simulink model "Fusion_Frame_Model_Architecture"  (R2018a)
settings: Solver=FixedStepAuto  StartTime=0.0  StopTime=SimulationTime  FixedStep=SamplingTime  RelTol=1e-3
undefined symbols (not defined in the file or in its folder): ACTIVATE_CAM, ACTIVATE_RAD, CAM1_detTimeStamp, CAM1_MeasNoise, CAM1_objClassID, CAM1_PX, CAM1_PY, CAM1_VX, CAM1_VY, CAM2_detTimeStamp, CAM2_MeasNoise, CAM2_objClassID, CAM2_PX, CAM2_PY, CAM2_VX, CAM2_VY, CAM3_detTimeStamp, CAM3_MeasNoise, CAM3_objClassID, CAM3_PX, CAM3_PY, CAM3_VX, CAM3_VY, CAM4_detTimeStamp, CAM4_MeasNoise, CAM4_objClassID, CAM4_PX, CAM4_PY, CAM4_VX, CAM4_VY, CAM5_detTimeStamp, CAM5_MeasNoise, CAM5_objClassID, CAM5_PX, CAM5_PY, CAM5_VX, CAM5_VY, CAM6_detTimeStamp, CAM6_MeasNoise, CAM6_objClassID, CAM6_PX, CAM6_PY, CAM6_VX, CAM6_VY, CAM7_detTimeStamp, CAM7_MeasNoise, CAM7_objClassID, CAM7_PX, CAM7_PY, CAM7_VX, CAM7_VY, CAM8_detTimeStamp, CAM8_MeasNoise, CAM8_objClassID, CAM8_PX, CAM8_PY, CAM8_VX, CAM8_VY, CAM_nMeas, CAM_TYPE ... (+181)
libraries: simulink_extras x4
(part 1 of 11)
settings Model: SimulationMode=accelerator  Creator=Udit Bhaskar  LastModifiedBy=Udit Bhaskar
settings OptimizationCC: EfficientMapNaN2IntZero=off
settings HardwareCC: TargetBitPerPointer=64  TargetBitPerSizeT=64  TargetBitPerPtrDiffT=64  TargetLongLongMode=on  TargetIntDivRoundTo=Zero  TargetEndianess=LittleEndian  TargetWordSize=64  TargetHWDeviceType=MATLAB Host  ProdEqTarget=off
settings CodeAppCC: MaxIdLength=128
settings GRTTargetCC: TargetLangStandard=C89/C90 (ANSI)  CombineOutputUpdateFcns=off  GRTInterface=on

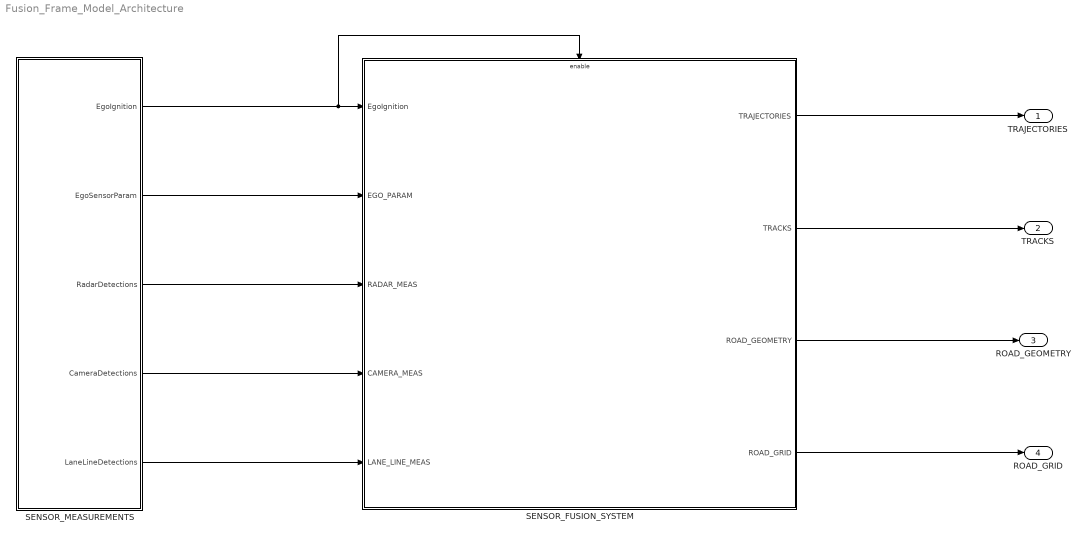
== system Fusion_Frame_Model_Architecture ==
  SENSOR_FUSION_SYSTEM : Subsystem
  SENSOR_MEASUREMENTS : Subsystem
  TRAJECTORIES : Outport
  TRACKS : Outport  Port=2
  ROAD_GEOMETRY : Outport  Port=3
  ROAD_GRID : Outport  Port=4
  wires:
  SENSOR_MEASUREMENTS/2(EgoSensorParam) -> SENSOR_FUSION_SYSTEM/2(EGO_PARAM)
  SENSOR_MEASUREMENTS/3(RadarDetections) -> SENSOR_FUSION_SYSTEM/3(RADAR_MEAS)
  SENSOR_MEASUREMENTS/4(CameraDetections) -> SENSOR_FUSION_SYSTEM/4(CAMERA_MEAS)
  SENSOR_MEASUREMENTS/5(LaneLineDetections) -> SENSOR_FUSION_SYSTEM/5(LANE_LINE_MEAS)
  SENSOR_FUSION_SYSTEM/2(TRACKS) -> TRACKS/1
  SENSOR_FUSION_SYSTEM/4(ROAD_GRID) -> ROAD_GRID/1
  SENSOR_FUSION_SYSTEM/1(TRAJECTORIES) -> TRAJECTORIES/1
  SENSOR_FUSION_SYSTEM/3(ROAD_GEOMETRY) -> ROAD_GEOMETRY/1
  SENSOR_MEASUREMENTS/1(EgoIgnition) -> SENSOR_FUSION_SYSTEM/1(EgoIgnition), SENSOR_FUSION_SYSTEM/Enable

== system Fusion_Frame_Model_Architecture/SENSOR_FUSION_SYSTEM ==
  EgoIgnition : Inport
  EGO_PARAM : Inport  Port=2
  RADAR_MEAS : Inport  Port=3
  CAMERA_MEAS : Inport  Port=4
  LANE_LINE_MEAS : Inport  Port=5
  Enable : EnablePort
  OBJECT_TRACKER_SENSOR_FUSION : Subsystem
  ROAD_GEOMETRY_CAMERA_FUSION : Subsystem
  Terminator : Terminator
  TRAJECTORIES : Outport
  TRACKS : Outport  Port=2
  ROAD_GEOMETRY : Outport  Port=3
  ROAD_GRID : Outport  Port=4
  wires:
  RADAR_MEAS/1 -> OBJECT_TRACKER_SENSOR_FUSION/3(RadCAN)
  LANE_LINE_MEAS/1 -> ROAD_GEOMETRY_CAMERA_FUSION/3(LINE_MEAS)
  OBJECT_TRACKER_SENSOR_FUSION/4(CamParam) -> ROAD_GEOMETRY_CAMERA_FUSION/1(CAM_SNSR_PARAM)
  [ego] -> ROAD_GEOMETRY_CAMERA_FUSION/2(EGO_PARAM)
  EGO_PARAM/1 -> [ego], OBJECT_TRACKER_SENSOR_FUSION/2(EgoData)
  CAMERA_MEAS/1 -> OBJECT_TRACKER_SENSOR_FUSION/4(CamCAN)
  EgoIgnition/1 -> OBJECT_TRACKER_SENSOR_FUSION/1(EgoIgnition)
  OBJECT_TRACKER_SENSOR_FUSION/1("TRAJECTORY_DATA ") -> TRAJECTORIES/1
  OBJECT_TRACKER_SENSOR_FUSION/2(TRACK_DATA) -> TRACKS/1
  ROAD_GEOMETRY_CAMERA_FUSION/1(ROAD_GEOMETRY) -> ROAD_GEOMETRY/1
  ROAD_GEOMETRY_CAMERA_FUSION/2(ROAD_GRID) -> ROAD_GRID/1
  OBJECT_TRACKER_SENSOR_FUSION/3(SENSOR_FOV_GRID) -> Terminator/1

== system Fusion_Frame_Model_Architecture/SENSOR_MEASUREMENTS ==
  RADAR_CAMERA_EGO_SENSOR_INTERFACE : Subsystem
  Subsystem : Subsystem
  Subsystem1 : Subsystem
  EgoIgnition : Outport
  EgoSensorParam : Outport  Port=2
  RadarDetections : Outport  Port=3
  CameraDetections : Outport  Port=4
  LaneLineDetections : Outport  Port=5
  wires:
  RADAR_CAMERA_EGO_SENSOR_INTERFACE/11(C5) -> Subsystem/11(C5)
  RADAR_CAMERA_EGO_SENSOR_INTERFACE/4(R4) -> Subsystem/4(R4)
  RADAR_CAMERA_EGO_SENSOR_INTERFACE/2(R2) -> Subsystem/2(R2)
  RADAR_CAMERA_EGO_SENSOR_INTERFACE/5(R5) -> Subsystem/5(R5)
  RADAR_CAMERA_EGO_SENSOR_INTERFACE/6(R6) -> Subsystem/6(R6)
  RADAR_CAMERA_EGO_SENSOR_INTERFACE/1(R1) -> Subsystem/1(R1)
  Subsystem/1(RadarMeasurementCAN) -> RadarDetections/1
  RADAR_CAMERA_EGO_SENSOR_INTERFACE/9(C3) -> Subsystem/9(C3)
  RADAR_CAMERA_EGO_SENSOR_INTERFACE/8(C2) -> Subsystem/8(C2)
  RADAR_CAMERA_EGO_SENSOR_INTERFACE/3(R3) -> Subsystem/3(R3)
  RADAR_CAMERA_EGO_SENSOR_INTERFACE/13(C7) -> Subsystem/13(C7)
  RADAR_CAMERA_EGO_SENSOR_INTERFACE/7(C1) -> Subsystem/7(C1)
  RADAR_CAMERA_EGO_SENSOR_INTERFACE/10(C4) -> Subsystem/10(C4)
  RADAR_CAMERA_EGO_SENSOR_INTERFACE/12(C6) -> Subsystem/12(C6)
  Subsystem/2(CameraMeasurementCAN) -> CameraDetections/1
  RADAR_CAMERA_EGO_SENSOR_INTERFACE/14(C8) -> Subsystem/14(C8)
  RADAR_CAMERA_EGO_SENSOR_INTERFACE/15(CAM_LINE1) -> Subsystem1/1(CAM_LINE1)
  RADAR_CAMERA_EGO_SENSOR_INTERFACE/16(CAM_LINE2) -> Subsystem1/2(CAM_LINE2)
  RADAR_CAMERA_EGO_SENSOR_INTERFACE/17(CAM_LINE3) -> Subsystem1/3(CAM_LINE3)
  RADAR_CAMERA_EGO_SENSOR_INTERFACE/18(CAM_LINE4) -> Subsystem1/4(CAM_LINE4)
  RADAR_CAMERA_EGO_SENSOR_INTERFACE/19(CAM_LINE5) -> Subsystem1/5(CAM_LINE5)
  RADAR_CAMERA_EGO_SENSOR_INTERFACE/20(CAM_LINE6) -> Subsystem1/6(CAM_LINE6)
  RADAR_CAMERA_EGO_SENSOR_INTERFACE/21(CAM_LINE7) -> Subsystem1/7(CAM_LINE7)
  RADAR_CAMERA_EGO_SENSOR_INTERFACE/22(CAM_LINE8) -> Subsystem1/8(CAM_LINE8)
  Subsystem1/1(LineMeasurementsCAN) -> LaneLineDetections/1
  RADAR_CAMERA_EGO_SENSOR_INTERFACE/23(EGO) -> EgoSensorParam/1
  RADAR_CAMERA_EGO_SENSOR_INTERFACE/24(EgoIgnition) -> EgoIgnition/1

== system Fusion_Frame_Model_Architecture/SENSOR_FUSION_SYSTEM/OBJECT_TRACKER_SENSOR_FUSION ==
  EgoIgnition : Inport
  EgoData : Inport  Port=2
  RadCAN : Inport  Port=3
  CamCAN : Inport  Port=4
  CAMERA_HOMOGENEOUS_FUSION : Subsystem
  RADAR_CAMERA_HETEROGENEOUS_FUSION : Subsystem
  RADAR_HOMOGENEOUS_FUSION : Subsystem
  SENSOR_LAYOUT_AND_CHRACTERIZATION : Subsystem
  SPATIAL_ALLIGNMENT1 : Subsystem
  TRACKS_TRAJECTORY_COMPUTATION : Subsystem
  Unit Delay : UnitDelay  InitialCondition=false  SampleTime=-1
  "TRAJECTORY_DATA " : Outport
  TRACK_DATA : Outport  Port=2
  SENSOR_FOV_GRID : Outport  Port=3
  CamParam : Outport  Port=4
  wires:
  EgoData/1 -> TRACKS_TRAJECTORY_COMPUTATION/2(EGO_DATA)
  SPATIAL_ALLIGNMENT1/1(RadarMeasTransformed) -> RADAR_HOMOGENEOUS_FUSION/3(RADAR_MEAS)
  RadCAN/1 -> SPATIAL_ALLIGNMENT1/3(RadarCAN)
  SPATIAL_ALLIGNMENT1/2(CameraMeasTransformed) -> CAMERA_HOMOGENEOUS_FUSION/2(CAMERA_MEAS)
  CamCAN/1 -> SPATIAL_ALLIGNMENT1/4(CameraCAN)
  SENSOR_LAYOUT_AND_CHRACTERIZATION/1(RAD_SNSR_PARAM) -> SPATIAL_ALLIGNMENT1/1(RadarCallibrationParam), [RAD_PARAM]
  SENSOR_LAYOUT_AND_CHRACTERIZATION/2(CAM_SNSR_PARAM) -> SPATIAL_ALLIGNMENT1/2(CameraCallibrationParam), [CAM_PARAM]
  SENSOR_LAYOUT_AND_CHRACTERIZATION/3(GRID_CHARACTERIZATION) -> [GRID]
  EgoIgnition/1 -> Unit Delay/1
  Unit Delay/1 -> SENSOR_LAYOUT_AND_CHRACTERIZATION/Trigger
  [GRID] -> CAMERA_HOMOGENEOUS_FUSION/1(GRID), RADAR_HOMOGENEOUS_FUSION/4(GRID)
  RADAR_HOMOGENEOUS_FUSION/1(RADAR_TRACKS_FUS) -> RADAR_CAMERA_HETEROGENEOUS_FUSION/1(RADAR_TRACKS_FUS), RADAR_HOMOGENEOUS_FUSION/1(RADAR_TRACKS_PREV)
  CAMERA_HOMOGENEOUS_FUSION/1(CAMERA_TRACKS_FUS) -> RADAR_CAMERA_HETEROGENEOUS_FUSION/2(CAMERA_TRACKS_FUS), CAMERA_HOMOGENEOUS_FUSION/4(CAMERA_TRACKS_PREV)
  TRACKS_TRAJECTORY_COMPUTATION/1(TRAJECTORY) -> "TRAJECTORY_DATA "/1, TRACKS_TRAJECTORY_COMPUTATION/1(TRAJECTORIES_PREV)
  [RAD_PARAM] -> RADAR_HOMOGENEOUS_FUSION/2(RAD_PARAM)
  [CAM_PARAM] -> CAMERA_HOMOGENEOUS_FUSION/3(CAM_PARAM)
  RADAR_CAMERA_HETEROGENEOUS_FUSION/1(FUS_TRACKS) -> TRACKS_TRAJECTORY_COMPUTATION/3(RAD_CAM_TRACKS_FUS), TRACK_DATA/1, RADAR_CAMERA_HETEROGENEOUS_FUSION/3(RAD_CAM_TRACKS_PREV)
  [GRID] -> SENSOR_FOV_GRID/1
  [CAM_PARAM] -> CamParam/1

== system Fusion_Frame_Model_Architecture/SENSOR_FUSION_SYSTEM/ROAD_GEOMETRY_CAMERA_FUSION ==
  CAM_SNSR_PARAM : Inport
  EGO_PARAM : Inport  Port=2
  LINE_MEAS : Inport  Port=3
  EGO_LANE_CENTER_LINE_ESTIMATION_FROM_LEFT_BOUNDARY : Subsystem
  EGO_LANE_CENTER_LINE_ESTIMATION_FROM_RIGHT_BOUNDARY : Subsystem
  EGO_LANE_CENTER_LINE_HYPOTHESIS_FUSION : Subsystem
  EGO_LANE_LEFT_BOUNDARY_LINE_FUSION : Subsystem
  EGO_LANE_RIGHT_BOUNDARY_LINE_FUSION : Subsystem
  EGO_LANE_WIDTH_ESTIMATION : Subsystem
  ROAD_GEOMERY_AND_GRID_COMPUTATION : Subsystem
  SPATIAL_ALLIGNMENT_CLOTHOID_COEFFICIENTS : Subsystem
  ROAD_GEOMETRY : Outport
  ROAD_GRID : Outport  Port=2
  wires:
  LINE_MEAS/1 -> SPATIAL_ALLIGNMENT_CLOTHOID_COEFFICIENTS/2(LINE_CLOTHOID_MEASUREMENTS)
  EGO_LANE_LEFT_BOUNDARY_LINE_FUSION/1(EGO_LANE_LEFT_LINE_TRACK) -> EGO_LANE_WIDTH_ESTIMATION/2(EGO_LANE_RIGHT_LINE_TRACK), EGO_LANE_LEFT_BOUNDARY_LINE_FUSION/1(EGO_LANE_LEFT_LINE_TRACK_prev), EGO_LANE_CENTER_LINE_ESTIMATION_FROM_LEFT_BOUNDARY/2(EGO_LANE_LEFT_LINE_TRACK)
  EGO_LANE_CENTER_LINE_HYPOTHESIS_FUSION/1(EGO_LANE_CENTER_LINE_CURR) -> ROAD_GEOMERY_AND_GRID_COMPUTATION/2(EGO_LANE_CENTER_LINE_TRACK)
  CAM_SNSR_PARAM/1 -> SPATIAL_ALLIGNMENT_CLOTHOID_COEFFICIENTS/1(CAM_SENSOR_PARAM)
  SPATIAL_ALLIGNMENT_CLOTHOID_COEFFICIENTS/1(LEFT_LINE_MEAS) -> EGO_LANE_LEFT_BOUNDARY_LINE_FUSION/2(EGO_LANE_LEFT_LINE_MEAS)
  EGO_LANE_RIGHT_BOUNDARY_LINE_FUSION/1(EGO_LANE_RIGHT_LINE_TRACK) -> EGO_LANE_WIDTH_ESTIMATION/3(EGO_LANE_LEFT_LINE_TRACK), EGO_LANE_CENTER_LINE_ESTIMATION_FROM_RIGHT_BOUNDARY/2(EGO_LANE_RIGHT_LINE_TRACK), EGO_LANE_RIGHT_BOUNDARY_LINE_FUSION/2(EGO_LANE_RIGHT_LINE_TRACK_prev)
  EGO_LANE_WIDTH_ESTIMATION/1(EGO_LANE_WIDTH) -> EGO_LANE_WIDTH_ESTIMATION/1(EGO_LANE_WIDTH_prev), EGO_LANE_CENTER_LINE_ESTIMATION_FROM_LEFT_BOUNDARY/3(EGO_LANE_WIDTH), EGO_LANE_CENTER_LINE_ESTIMATION_FROM_RIGHT_BOUNDARY/1(EGO_LANE_WIDTH), [WIDTH]
  EGO_LANE_CENTER_LINE_ESTIMATION_FROM_LEFT_BOUNDARY/1(EGO_LANE_CENTER_LINE_TRACK_HYP1) -> EGO_LANE_CENTER_LINE_HYPOTHESIS_FUSION/1(EGO_LANE_CENTER_LINE_HYP1)
  ROAD_GEOMERY_AND_GRID_COMPUTATION/2(ROAD_GRID) -> ROAD_GRID/1, ROAD_GEOMERY_AND_GRID_COMPUTATION/4(ROAD_GRID_prev)
  EGO_PARAM/1 -> [EGO_PARAM]
  [WIDTH] -> ROAD_GEOMERY_AND_GRID_COMPUTATION/1(EGO_LANE_WIDTH)
  [EGO_PARAM] -> ROAD_GEOMERY_AND_GRID_COMPUTATION/3(EGO_PARAM)
  ROAD_GEOMERY_AND_GRID_COMPUTATION/1(ROAD_GEOMETRY) -> ROAD_GEOMETRY/1
  SPATIAL_ALLIGNMENT_CLOTHOID_COEFFICIENTS/2("RIGHT_LINE_MEAS ") -> EGO_LANE_RIGHT_BOUNDARY_LINE_FUSION/1(EGO_LANE_RIGHT_LINE_MEAS)
  EGO_LANE_CENTER_LINE_ESTIMATION_FROM_RIGHT_BOUNDARY/1(EGO_LANE_CENTER_LINE_TRACK_HYP2) -> EGO_LANE_CENTER_LINE_HYPOTHESIS_FUSION/2(EGO_LANE_CENTER_LINE_HYP2)
  EGO_LANE_CENTER_LINE_HYPOTHESIS_FUSION/2(EGO_LANE_CENTER_LINE_PRED) -> EGO_LANE_CENTER_LINE_ESTIMATION_FROM_RIGHT_BOUNDARY/3(EGO_LANE_CENTER_LINE_TRACK_pred), EGO_LANE_CENTER_LINE_ESTIMATION_FROM_LEFT_BOUNDARY/1(EGO_LANE_CENTER_LINE_TRACK_pred)

== system Fusion_Frame_Model_Architecture/SENSOR_MEASUREMENTS/RADAR_CAMERA_EGO_SENSOR_INTERFACE ==
  CameraSensors : Subsystem
  Clock : Subsystem
  EgoSensors : Subsystem
  Ground{,1..3} (4 alike) : Ground
  RadarSensors : Subsystem
  RoadSensors : Subsystem
  R1 : Outport
  R2 : Outport  Port=2
  R3 : Outport  Port=3
  R4 : Outport  Port=4
  R5 : Outport  Port=5
  R6 : Outport  Port=6
  C1 : Outport  Port=7
  C2 : Outport  Port=8
  C3 : Outport  Port=9
  C4 : Outport  Port=10
  C5 : Outport  Port=11
  C6 : Outport  Port=12
  C7 : Outport  Port=13
  C8 : Outport  Port=14
  CAM_LINE1 : Outport  Port=15
  CAM_LINE2 : Outport  Port=16
  CAM_LINE3 : Outport  Port=17
  CAM_LINE4 : Outport  Port=18
  CAM_LINE5 : Outport  Port=19
  CAM_LINE6 : Outport  Port=20
  CAM_LINE7 : Outport  Port=21
  CAM_LINE8 : Outport  Port=22
  EGO : Outport  Port=23
  EgoIgnition : Outport  Port=24
  wires:
  RadarSensors/6(R6) -> R6/1
  RadarSensors/4(R4) -> R4/1
  Clock/2(nObjRadar) -> RadarSensors/2(nObjRadar)
  Clock/3(nObjCamera) -> CameraSensors/2(nObjCamera)
  CameraSensors/3(C3) -> C3/1
  RadarSensors/5(R5) -> R5/1
  CameraSensors/5(C5) -> C5/1
  CameraSensors/4(C4) -> C4/1
  CameraSensors/8(C8) -> C8/1
  CameraSensors/7(C7) -> C7/1
  CameraSensors/6(C6) -> C6/1
  CameraSensors/2(C2) -> C2/1
  RadarSensors/2(R2) -> R2/1
  RadarSensors/3(R3) -> R3/1
  CameraSensors/1(C1) -> C1/1
  RadarSensors/1(R1) -> R1/1
  Clock/1(time) -> CameraSensors/1(time), RoadSensors/1(time), EgoSensors/1(timeIdx), RadarSensors/1(time)
  Clock/4(nLinesCamera) -> RoadSensors/2(nLinesCamera)
  RoadSensors/1(C1) -> CAM_LINE1/1
  RoadSensors/2(C2) -> CAM_LINE2/1
  RoadSensors/3(C3) -> CAM_LINE3/1
  RoadSensors/4(C4) -> CAM_LINE4/1
  RoadSensors/5(C5) -> CAM_LINE5/1
  RoadSensors/6(C6) -> CAM_LINE6/1
  RoadSensors/7(C7) -> CAM_LINE7/1
  RoadSensors/8(C8) -> CAM_LINE8/1
  EgoSensors/1(EgoSensorData) -> EGO/1
  Ground1/1 -> RadarSensors/3(RADSensorBUS)
  Ground2/1 -> CameraSensors/3(CAMSensorBUS)
  Ground/1 -> EgoSensors/2(In1)
  Ground3/1 -> RoadSensors/3(CameraLineCoeff1)
  EgoSensors/2(EgoIgnitionStatus) -> EgoIgnition/1

== system Fusion_Frame_Model_Architecture/SENSOR_MEASUREMENTS/Subsystem ==
  R1 : Inport
  R2 : Inport  Port=2
  R3 : Inport  Port=3
  R4 : Inport  Port=4
  R5 : Inport  Port=5
  R6 : Inport  Port=6
  C1 : Inport  Port=7
  C2 : Inport  Port=8
  C3 : Inport  Port=9
  C4 : Inport  Port=10
  C5 : Inport  Port=11
  C6 : Inport  Port=12
  C7 : Inport  Port=13
  C8 : Inport  Port=14
  Bus Creator : BusCreator  Inputs=6  OutDataTypeStr=Bus: RAD_MEAS_INTERFACE  NonVirtualBus=on
      settings: InheritFromInputs=off
  Bus Creator1 : BusCreator  Inputs=8  OutDataTypeStr=Bus: CAM_MEAS_INTERFACE  NonVirtualBus=on
      settings: InheritFromInputs=off
  RadarMeasurementCAN : Outport
  CameraMeasurementCAN : Outport  Port=2
  wires:
  R1/1 -> Bus Creator/1  "R1"
  R6/1 -> Bus Creator/6  "R6"
  R5/1 -> Bus Creator/5  "R5"
  R4/1 -> Bus Creator/4  "R4"
  R3/1 -> Bus Creator/3  "R3"
  R2/1 -> Bus Creator/2  "R2"
  Bus Creator/1 -> RadarMeasurementCAN/1
  C1/1 -> Bus Creator1/1  "C1"
  C2/1 -> Bus Creator1/2  "C2"
  C3/1 -> Bus Creator1/3  "C3"
  C4/1 -> Bus Creator1/4  "C4"
  C5/1 -> Bus Creator1/5  "C5"
  C6/1 -> Bus Creator1/6  "C6"
  C7/1 -> Bus Creator1/7  "C7"
  C8/1 -> Bus Creator1/8  "C8"
  Bus Creator1/1 -> CameraMeasurementCAN/1

== system Fusion_Frame_Model_Architecture/SENSOR_MEASUREMENTS/Subsystem1 ==
  CAM_LINE1 : Inport
  CAM_LINE2 : Inport  Port=2
  CAM_LINE3 : Inport  Port=3
  CAM_LINE4 : Inport  Port=4
  CAM_LINE5 : Inport  Port=5
  CAM_LINE6 : Inport  Port=6
  CAM_LINE7 : Inport  Port=7
  CAM_LINE8 : Inport  Port=8
  Bus Creator : BusCreator  Inputs=8  OutDataTypeStr=Bus: LINE_MEAS_INTERFACE  NonVirtualBus=on
      settings: InheritFromInputs=off
  LineMeasurementsCAN : Outport
  wires:
  CAM_LINE1/1 -> Bus Creator/1  "C1_LINE"
  CAM_LINE2/1 -> Bus Creator/2  "C2_LINE"
  CAM_LINE3/1 -> Bus Creator/3  "C3_LINE"
  CAM_LINE4/1 -> Bus Creator/4  "C4_LINE"
  CAM_LINE5/1 -> Bus Creator/5  "C5_LINE"
  CAM_LINE6/1 -> Bus Creator/6  "C6_LINE"
  CAM_LINE7/1 -> Bus Creator/7  "C7_LINE"
  CAM_LINE8/1 -> Bus Creator/8  "C8_LINE"
  Bus Creator/1 -> LineMeasurementsCAN/1

== system Fusion_Frame_Model_Architecture/SENSOR_FUSION_SYSTEM/OBJECT_TRACKER_SENSOR_FUSION/CAMERA_HOMOGENEOUS_FUSION ==
  GRID : Inport
  CAMERA_MEAS : Inport  Port=2
  CAM_PARAM : Inport  Port=3
  CAMERA_TRACKS_PREV : Inport  Port=4
  DATA_ASSOCIATION_AND_ESTIMATION : Subsystem
  GATING : Subsystem
  NEAREST_NEIGHBOUR_CLUSTERING_FOR_CAMERA_MEASUREMENT : Subsystem
  STATE_PREDICTION : Subsystem
  TRACK_MANAGER : Subsystem
  CAMERA_TRACKS_FUS : Outport
  wires:
  CAMERA_MEAS/1 -> GATING/1(MEAS), [CAM_MEAS], NEAREST_NEIGHBOUR_CLUSTERING_FOR_CAMERA_MEASUREMENT/1(CAMERA_MEAS)
  NEAREST_NEIGHBOUR_CLUSTERING_FOR_CAMERA_MEASUREMENT/1(CAMERA_CLUSTERS) -> GATING/2(CAMERA_CLUSTERS)
  DATA_ASSOCIATION_AND_ESTIMATION/1(TrackParamUpd) -> TRACK_MANAGER/1(TrackParamIn)
  STATE_PREDICTION/1(TrackParamPred) -> GATING/4(TrackParamPred), DATA_ASSOCIATION_AND_ESTIMATION/5(TrackParamPred)
  [unGatedClstr] -> TRACK_MANAGER/2(UnGatedClusters)
  GATING/1(GatedMeasFlag) -> DATA_ASSOCIATION_AND_ESTIMATION/1(GatedMeasFlag)
  GRID/1 -> TRACK_MANAGER/3(Grid)
  GATING/2(GatedMeasLogLikelihood) -> DATA_ASSOCIATION_AND_ESTIMATION/2(MeasLogLikelihood)
  [CAM_MEAS] -> DATA_ASSOCIATION_AND_ESTIMATION/3(Meas)
  GATING/3(UnGatedMeasCluster) -> [unGatedClstr]
  CAMERA_TRACKS_PREV/1 -> STATE_PREDICTION/1(TrackParamPrev)
  TRACK_MANAGER/1(TrackParamUpd) -> CAMERA_TRACKS_FUS/1
  CAM_PARAM/1 -> [CAM_PARAM]
  [CAM_PARAM] -> GATING/3(CAM_PARAM)
  [CAM_PARAM] -> DATA_ASSOCIATION_AND_ESTIMATION/4(CAM_PARAM)

== system Fusion_Frame_Model_Architecture/SENSOR_FUSION_SYSTEM/OBJECT_TRACKER_SENSOR_FUSION/RADAR_CAMERA_HETEROGENEOUS_FUSION ==
  RADAR_TRACKS_FUS : Inport
  CAMERA_TRACKS_FUS : Inport  Port=2
  RAD_CAM_TRACKS_PREV : Inport  Port=3
  FORM_TRACK_GROUPS : Subsystem
  STATE_PREDICTION : Subsystem
  TRACK_MANAGER : Subsystem
  TRACK_TO_TRACK_FUSION : Subsystem
  FUS_TRACKS : Outport
  wires:
  RAD_CAM_TRACKS_PREV/1 -> [RAD_TRACKS], STATE_PREDICTION/1(RAD_CAM_TRACKS_PREV)
  STATE_PREDICTION/1(RAD_CAM_TRACKS_PRED) -> FORM_TRACK_GROUPS/2(RAD_CAM_FUSED_TRACKS), [FUSED_TRACKS]
  CAMERA_TRACKS_FUS/1 -> [CAM_TRACKS], FORM_TRACK_GROUPS/3(CAM_TRACKS)
  RADAR_TRACKS_FUS/1 -> FORM_TRACK_GROUPS/1(RAD_TRACKS)
  FORM_TRACK_GROUPS/1(GROUPED_TRACKS_IDs) -> TRACK_TO_TRACK_FUSION/1(GROUPED_TRACKS_IDs)
  TRACK_TO_TRACK_FUSION/1(RAD_CAM_FUSED_TRACKS_UPD) -> TRACK_MANAGER/1(RAD_CAM_FUSED_TRACKS)
  [CAM_TRACKS] -> TRACK_TO_TRACK_FUSION/3(CAM_TRACKS)
  [RAD_TRACKS] -> TRACK_TO_TRACK_FUSION/2(RAD_TRACKS)
  [FUSED_TRACKS] -> TRACK_TO_TRACK_FUSION/4(RAD_CAM_FUSED_TRACKS_PRED)
  [RAD_TRACKS] -> TRACK_MANAGER/2(RAD_TRACKS)
  [CAM_TRACKS] -> TRACK_MANAGER/3(CAM_TRACKS)
  TRACK_MANAGER/1(RAD_CAM_TRACKS_FUS) -> FUS_TRACKS/1

== system Fusion_Frame_Model_Architecture/SENSOR_FUSION_SYSTEM/OBJECT_TRACKER_SENSOR_FUSION/RADAR_HOMOGENEOUS_FUSION ==
  RADAR_TRACKS_PREV : Inport
  RAD_PARAM : Inport  Port=2
  RADAR_MEAS : Inport  Port=3
  GRID : Inport  Port=4
  DATA_ASSOCIATION_AND_ESTIMATION : Subsystem
  GATING : Subsystem
  SEGREGATE_CLUSTER : Subsystem
  SIMPLYFIED_DBSCAN_FOR_RADAR_MEASUREMENT_GROUPING : Subsystem
  STATE_PREDICTION : Subsystem
  TRACK_MANAGER : Subsystem
  RADAR_TRACKS_FUS : Outport
  wires:
  GRID/1 -> TRACK_MANAGER/3(Grid)
  RADAR_MEAS/1 -> SEGREGATE_CLUSTER/1(RADAR_MEAS), SIMPLYFIED_DBSCAN_FOR_RADAR_MEASUREMENT_GROUPING/1(RADAR_MEAS)
  SIMPLYFIED_DBSCAN_FOR_RADAR_MEASUREMENT_GROUPING/1(RADAR_CLUSTERS) -> SEGREGATE_CLUSTER/2(RADAR_CLUSTERS), GATING/3(RADAR_CLUSTERS)
  SEGREGATE_CLUSTER/1(RADAR_CLSTR_MEAS) -> GATING/1(MEAS), [RAD_MEAS]
  GATING/1(GatedMeasFlag) -> DATA_ASSOCIATION_AND_ESTIMATION/1(GatedMeasFlag)
  STATE_PREDICTION/1(TrackParamPred) -> GATING/4(TrackParamPred), DATA_ASSOCIATION_AND_ESTIMATION/5(TrackParamPred)
  GATING/2(GatedMeasLogLikelihood) -> DATA_ASSOCIATION_AND_ESTIMATION/2(MeasLogLikelihood)
  [RAD_MEAS] -> DATA_ASSOCIATION_AND_ESTIMATION/3(Meas)
  GATING/3(UnGatedMeasCluster) -> [unGatedClstr]
  DATA_ASSOCIATION_AND_ESTIMATION/1(TrackParamUpd) -> TRACK_MANAGER/1(TrackParamIn)
  [unGatedClstr] -> TRACK_MANAGER/2(UnGatedClusters)
  TRACK_MANAGER/1(TrackParamUpd) -> RADAR_TRACKS_FUS/1
  RAD_PARAM/1 -> [RAD_PARAM]
  [RAD_PARAM] -> GATING/2(RAD_PARAM)
  [RAD_PARAM] -> DATA_ASSOCIATION_AND_ESTIMATION/4(RAD_PARAM)
  RADAR_TRACKS_PREV/1 -> STATE_PREDICTION/1(TrackParamPrev)

== system Fusion_Frame_Model_Architecture/SENSOR_FUSION_SYSTEM/OBJECT_TRACKER_SENSOR_FUSION/SENSOR_LAYOUT_AND_CHRACTERIZATION ==
  Trigger : TriggerPort  VariantControl=Variant  PortDimensions=1
  Ground1 : Ground
  Ground2 : Ground
  PRE_COMPUTE_SENSOR_FOV_GRID : Subsystem
  SET_SENSOR_CALLIBRATION_PARAMETER : Subsystem
  RAD_SNSR_PARAM : Outport
  CAM_SNSR_PARAM : Outport  Port=2
  GRID_CHARACTERIZATION : Outport  Port=3
  wires:
  SET_SENSOR_CALLIBRATION_PARAMETER/2(CameraCalibParamUpd) -> CAM_SNSR_PARAM/1, PRE_COMPUTE_SENSOR_FOV_GRID/2(CAMSnsrParam)
  Ground2/1 -> SET_SENSOR_CALLIBRATION_PARAMETER/2(RADSnsrParam)
  Ground1/1 -> SET_SENSOR_CALLIBRATION_PARAMETER/1(CamCalibParam)
  SET_SENSOR_CALLIBRATION_PARAMETER/1(RadarCalibParamUpd) -> RAD_SNSR_PARAM/1, PRE_COMPUTE_SENSOR_FOV_GRID/1(RADSnsrParam)
  PRE_COMPUTE_SENSOR_FOV_GRID/1(GRID_CHARACTERIZATION) -> GRID_CHARACTERIZATION/1

== system Fusion_Frame_Model_Architecture/SENSOR_FUSION_SYSTEM/OBJECT_TRACKER_SENSOR_FUSION/SPATIAL_ALLIGNMENT1 ==
  RadarCallibrationParam : Inport
  CameraCallibrationParam : Inport  Port=2
  RadarCAN : Inport  Port=3
  CameraCAN : Inport  Port=4
  CAMERA_MEASUREMENTS_SPATIAL_ALLIGNMENT : Subsystem
  GET_CAM_MEAS : Subsystem
  GET_RAD_MEAS : Subsystem
  RADAR_MEASUREMENTS_SPATIAL_ALLIGNMENT : Subsystem
  RadarMeasTransformed : Outport
  CameraMeasTransformed : Outport  Port=2
  wires:
  RadarCAN/1 -> GET_RAD_MEAS/2(RadarMeas)
  CameraCAN/1 -> GET_CAM_MEAS/2(CameraMeas)
  GET_CAM_MEAS/2(<C1>) -> CAMERA_MEASUREMENTS_SPATIAL_ALLIGNMENT/2(C1)
  GET_CAM_MEAS/3(<C2>) -> CAMERA_MEASUREMENTS_SPATIAL_ALLIGNMENT/3(C2)
  GET_CAM_MEAS/4(<C3>) -> CAMERA_MEASUREMENTS_SPATIAL_ALLIGNMENT/4(C3)
  GET_CAM_MEAS/5(<C4>) -> CAMERA_MEASUREMENTS_SPATIAL_ALLIGNMENT/5(C4)
  GET_CAM_MEAS/6(<C5>) -> CAMERA_MEASUREMENTS_SPATIAL_ALLIGNMENT/6(C5)
  GET_CAM_MEAS/7(<C6>) -> CAMERA_MEASUREMENTS_SPATIAL_ALLIGNMENT/7(C6)
  GET_CAM_MEAS/8(<C7>) -> CAMERA_MEASUREMENTS_SPATIAL_ALLIGNMENT/8(C7)
  GET_CAM_MEAS/9(<C8>) -> CAMERA_MEASUREMENTS_SPATIAL_ALLIGNMENT/9(C8)
  GET_RAD_MEAS/2(<R1>) -> RADAR_MEASUREMENTS_SPATIAL_ALLIGNMENT/2(R1)
  GET_RAD_MEAS/3(<R2>) -> RADAR_MEASUREMENTS_SPATIAL_ALLIGNMENT/3(R2)
  GET_RAD_MEAS/4(<R3>) -> RADAR_MEASUREMENTS_SPATIAL_ALLIGNMENT/4(R3)
  GET_RAD_MEAS/5(<R4>) -> RADAR_MEASUREMENTS_SPATIAL_ALLIGNMENT/5(R4)
  GET_RAD_MEAS/6(<R5>) -> RADAR_MEASUREMENTS_SPATIAL_ALLIGNMENT/6(R5)
  GET_RAD_MEAS/7(<R6>) -> RADAR_MEASUREMENTS_SPATIAL_ALLIGNMENT/7(R6)
  GET_RAD_MEAS/1(SnsrParam) -> RADAR_MEASUREMENTS_SPATIAL_ALLIGNMENT/1(RadarCalibParam)
  RadarCallibrationParam/1 -> GET_RAD_MEAS/1(RadarParam)
  GET_CAM_MEAS/1(SnsrParam) -> CAMERA_MEASUREMENTS_SPATIAL_ALLIGNMENT/1(CameraCalibParam)
  CameraCallibrationParam/1 -> GET_CAM_MEAS/1(CameraParam)
  CAMERA_MEASUREMENTS_SPATIAL_ALLIGNMENT/1(CameraMeasTransformed) -> CameraMeasTransformed/1
  RADAR_MEASUREMENTS_SPATIAL_ALLIGNMENT/1(RadarMeasTransformed) -> RadarMeasTransformed/1

== system Fusion_Frame_Model_Architecture/SENSOR_FUSION_SYSTEM/OBJECT_TRACKER_SENSOR_FUSION/TRACKS_TRAJECTORY_COMPUTATION ==
  TRAJECTORIES_PREV : Inport
  EGO_DATA : Inport  Port=2
  RAD_CAM_TRACKS_FUS : Inport  Port=3
  EGO_COMPENSATE_TRAJECTORY_HISTORY_BUFFER : Subsystem
  UPDATE_TRAJECTORY_BUFFER_WITH_CURRENT_TRACK_DATA : Subsystem
  TRAJECTORY : Outport
  wires:
  EGO_DATA/1 -> EGO_COMPENSATE_TRAJECTORY_HISTORY_BUFFER/1(RAD_CAM_TRACKS_FUS)
  RAD_CAM_TRACKS_FUS/1 -> UPDATE_TRAJECTORY_BUFFER_WITH_CURRENT_TRACK_DATA/1(RAD_CAM_TRACKS_FUS)
  TRAJECTORIES_PREV/1 -> UPDATE_TRAJECTORY_BUFFER_WITH_CURRENT_TRACK_DATA/2(TRAJECTORIES)
  UPDATE_TRAJECTORY_BUFFER_WITH_CURRENT_TRACK_DATA/1(TRAJECTORIES_UPD) -> EGO_COMPENSATE_TRAJECTORY_HISTORY_BUFFER/2(TRAJECTORIES)
  EGO_COMPENSATE_TRAJECTORY_HISTORY_BUFFER/1(TRAJECTORIES_UPD) -> TRAJECTORY/1

== system Fusion_Frame_Model_Architecture/SENSOR_FUSION_SYSTEM/ROAD_GEOMETRY_CAMERA_FUSION/EGO_LANE_CENTER_LINE_ESTIMATION_FROM_LEFT_BOUNDARY ==
  EGO_LANE_CENTER_LINE_TRACK_pred : Inport
  EGO_LANE_LEFT_LINE_TRACK : Inport  Port=2
  EGO_LANE_WIDTH : Inport  Port=3
  CURVE_FITTING_BY_LEAST_SQUARES : Subsystem
  GENERATE_POINTS_AT_EGO_LANE_CENTER : Subsystem
  INTERPOLATE_POINTS_ALONG_THE_LINE : Subsystem
  KALMAN_FILTER_STATE_UPDATE : Subsystem
  POLYNOMIAL_TO_CLOTHOID_CONVERSION : Subsystem
  EGO_LANE_CENTER_LINE_TRACK_HYP1 : Outport
  wires:
  EGO_LANE_LEFT_LINE_TRACK/1 -> INTERPOLATE_POINTS_ALONG_THE_LINE/1(LEFT_LINE_TRACK)
  EGO_LANE_WIDTH/1 -> GENERATE_POINTS_AT_EGO_LANE_CENTER/2(EgoLaneWidth)
  EGO_LANE_CENTER_LINE_TRACK_pred/1 -> KALMAN_FILTER_STATE_UPDATE/2(CenterLinePred)
  INTERPOLATE_POINTS_ALONG_THE_LINE/1(PointsAlongTheLine) -> GENERATE_POINTS_AT_EGO_LANE_CENTER/1(PointsAlongTheLine)
  GENERATE_POINTS_AT_EGO_LANE_CENTER/1(PointsAlongEgoLaneCenter) -> CURVE_FITTING_BY_LEAST_SQUARES/1(Points)
  CURVE_FITTING_BY_LEAST_SQUARES/1(PolynomialCoefficients) -> POLYNOMIAL_TO_CLOTHOID_CONVERSION/1(PolynomialCoefficients)
  POLYNOMIAL_TO_CLOTHOID_CONVERSION/1(ClothoidCoefficients) -> KALMAN_FILTER_STATE_UPDATE/1(CenterLineHypothesis)
  KALMAN_FILTER_STATE_UPDATE/1(CenterLineHypUpd) -> EGO_LANE_CENTER_LINE_TRACK_HYP1/1

== system Fusion_Frame_Model_Architecture/SENSOR_FUSION_SYSTEM/ROAD_GEOMETRY_CAMERA_FUSION/EGO_LANE_CENTER_LINE_ESTIMATION_FROM_RIGHT_BOUNDARY ==
  EGO_LANE_WIDTH : Inport
  EGO_LANE_RIGHT_LINE_TRACK : Inport  Port=2
  EGO_LANE_CENTER_LINE_TRACK_pred : Inport  Port=3
  CURVE_FITTING_BY_LEAST_SQUARES : Subsystem
  GENERATE_POINTS_AT_EGO_LANE_CENTER : Subsystem
  INTERPOLATE_POINTS_ALONG_THE_LINE : Subsystem
  KALMAN_FILTER_STATE_UPDATE : Subsystem
  POLYNOMIAL_TO_CLOTHOID_CONVERSION : Subsystem
  EGO_LANE_CENTER_LINE_TRACK_HYP2 : Outport
  wires:
  INTERPOLATE_POINTS_ALONG_THE_LINE/1(PointsAlongTheLine) -> GENERATE_POINTS_AT_EGO_LANE_CENTER/1(PointsAlongTheLine)
  EGO_LANE_RIGHT_LINE_TRACK/1 -> INTERPOLATE_POINTS_ALONG_THE_LINE/1(LEFT_LINE_TRACK)
  CURVE_FITTING_BY_LEAST_SQUARES/1(PolynomialCoefficients) -> POLYNOMIAL_TO_CLOTHOID_CONVERSION/1(PolynomialCoefficients)
  GENERATE_POINTS_AT_EGO_LANE_CENTER/1(PointsAlongEgoLaneCenter) -> CURVE_FITTING_BY_LEAST_SQUARES/1(Points)
  KALMAN_FILTER_STATE_UPDATE/1(CenterLineHypUpd) -> EGO_LANE_CENTER_LINE_TRACK_HYP2/1
  POLYNOMIAL_TO_CLOTHOID_CONVERSION/1(ClothoidCoefficients) -> KALMAN_FILTER_STATE_UPDATE/1(CenterLineHypothesis)
  EGO_LANE_CENTER_LINE_TRACK_pred/1 -> KALMAN_FILTER_STATE_UPDATE/2(CenterLinePred)
  EGO_LANE_WIDTH/1 -> GENERATE_POINTS_AT_EGO_LANE_CENTER/2(EgoLaneWidth)

== system Fusion_Frame_Model_Architecture/SENSOR_FUSION_SYSTEM/ROAD_GEOMETRY_CAMERA_FUSION/EGO_LANE_CENTER_LINE_HYPOTHESIS_FUSION ==
  EGO_LANE_CENTER_LINE_HYP1 : Inport
  EGO_LANE_CENTER_LINE_HYP2 : Inport  Port=2
  EGO_LANE_CENTER_LINE_PREDICTION : Subsystem
  HYPOTHESIS_MERGE : Subsystem
  WEIGHTAGE_COMPUTATION : Subsystem
  EGO_LANE_CENTER_LINE_CURR : Outport
  EGO_LANE_CENTER_LINE_PRED : Outport  Port=2
  wires:
  EGO_LANE_CENTER_LINE_HYP1/1 -> HYPOTHESIS_MERGE/1(EGO_LANE_CENTER_LINE_HYP1), WEIGHTAGE_COMPUTATION/1(EGO_LANE_CENTER_LINE_HYP1)
  EGO_LANE_CENTER_LINE_HYP2/1 -> HYPOTHESIS_MERGE/3(EGO_LANE_CENTER_LINE_HYP2), WEIGHTAGE_COMPUTATION/2(EGO_LANE_CENTER_LINE_HYP2)
  WEIGHTAGE_COMPUTATION/1(weight) -> HYPOTHESIS_MERGE/2(weight)
  HYPOTHESIS_MERGE/1(EGO_LANE_CENTER_LINE) -> EGO_LANE_CENTER_LINE_CURR/1, EGO_LANE_CENTER_LINE_PREDICTION/1(EGO_LANE_CENTER_LINE)
  EGO_LANE_CENTER_LINE_PREDICTION/1(EGO_LANE_CENTER_LINE_PRED) -> EGO_LANE_CENTER_LINE_PRED/1

== system Fusion_Frame_Model_Architecture/SENSOR_FUSION_SYSTEM/ROAD_GEOMETRY_CAMERA_FUSION/EGO_LANE_LEFT_BOUNDARY_LINE_FUSION ==
  EGO_LANE_LEFT_LINE_TRACK_prev : Inport
  EGO_LANE_LEFT_LINE_MEAS : Inport  Port=2
  FIND_UNGATED_LINE_MEASUREMENTS : Subsystem
  LANE_LINE_MEASUREMENT_TO_TRACK_FUSION : Subsystem
  LANE_LINE_MEASUREMENT_TO_TRACK_GATING : Subsystem
  LANE_LINE_STATE_PREDICTION : Subsystem
  LINE_TRACK_MANAGER : Subsystem
  EGO_LANE_LEFT_LINE_TRACK : Outport
  wires:
  EGO_LANE_LEFT_LINE_MEAS/1 -> LINE_TRACK_MANAGER/3(Line_Measurements), LANE_LINE_MEASUREMENT_TO_TRACK_FUSION/3(EGO_LANE_LEFT_LINE_MEAS), [Meas], LANE_LINE_MEASUREMENT_TO_TRACK_GATING/2(EGO_LANE_LEFT_LINE_MEAS)
  EGO_LANE_LEFT_LINE_TRACK_prev/1 -> LANE_LINE_STATE_PREDICTION/1(TrackParamPrev)
  LANE_LINE_STATE_PREDICTION/1(TrackParamPred) -> [prediction], LANE_LINE_MEASUREMENT_TO_TRACK_GATING/1(TrackParamPred)
  LANE_LINE_MEASUREMENT_TO_TRACK_GATING/1(GatedMeasIndex) -> LANE_LINE_MEASUREMENT_TO_TRACK_FUSION/1(GatedMeasIndex), FIND_UNGATED_LINE_MEASUREMENTS/1(GatedMeasIndex)
  [prediction] -> LANE_LINE_MEASUREMENT_TO_TRACK_FUSION/2(TrackParamPred)
  [Meas] -> FIND_UNGATED_LINE_MEASUREMENTS/2(EGO_LANE_LEFT_LINE_MEAS)
  FIND_UNGATED_LINE_MEASUREMENTS/1(UnGatedMeasIndex) -> LINE_TRACK_MANAGER/1(UnGatedMeasIndex)
  LANE_LINE_MEASUREMENT_TO_TRACK_FUSION/1(TrackParamUpd) -> LINE_TRACK_MANAGER/2(TrackParamUpd_in)
  LINE_TRACK_MANAGER/1(TrackParamUpd) -> EGO_LANE_LEFT_LINE_TRACK/1

== system Fusion_Frame_Model_Architecture/SENSOR_FUSION_SYSTEM/ROAD_GEOMETRY_CAMERA_FUSION/EGO_LANE_RIGHT_BOUNDARY_LINE_FUSION ==
  EGO_LANE_RIGHT_LINE_MEAS : Inport
  EGO_LANE_RIGHT_LINE_TRACK_prev : Inport  Port=2
  FIND_UNGATED_LINE_MEASUREMENTS : Subsystem
  LANE_LINE_MEASUREMENT_TO_TRACK_FUSION : Subsystem
  LANE_LINE_MEASUREMENT_TO_TRACK_GATING : Subsystem
  LANE_LINE_STATE_PREDICTION : Subsystem
  LINE_TRACK_MANAGER : Subsystem
  EGO_LANE_RIGHT_LINE_TRACK : Outport
  wires:
  LANE_LINE_MEASUREMENT_TO_TRACK_FUSION/1(TrackParamUpd) -> LINE_TRACK_MANAGER/2(TrackParamUpd_in)
  LANE_LINE_STATE_PREDICTION/1(TrackParamPred) -> [prediction], LANE_LINE_MEASUREMENT_TO_TRACK_GATING/1(TrackParamPred)
  EGO_LANE_RIGHT_LINE_MEAS/1 -> LINE_TRACK_MANAGER/3(Line_Measurements), LANE_LINE_MEASUREMENT_TO_TRACK_FUSION/3(EGO_LANE_RIGHT_LINE_MEAS), [Meas], LANE_LINE_MEASUREMENT_TO_TRACK_GATING/2(EGO_LANE_RIGHT_LINE_MEAS)
  LANE_LINE_MEASUREMENT_TO_TRACK_GATING/1(GatedMeasIndex) -> LANE_LINE_MEASUREMENT_TO_TRACK_FUSION/1(GatedMeasIndex), FIND_UNGATED_LINE_MEASUREMENTS/1(GatedMeasIndex)
  [Meas] -> FIND_UNGATED_LINE_MEASUREMENTS/2(EGO_LANE_RIGHT_LINE_MEAS)
  EGO_LANE_RIGHT_LINE_TRACK_prev/1 -> LANE_LINE_STATE_PREDICTION/1(TrackParamPrev)
  LINE_TRACK_MANAGER/1(TrackParamUpd) -> EGO_LANE_RIGHT_LINE_TRACK/1
  [prediction] -> LANE_LINE_MEASUREMENT_TO_TRACK_FUSION/2(TrackParamPred)
  FIND_UNGATED_LINE_MEASUREMENTS/1(UnGatedMeasIndex) -> LINE_TRACK_MANAGER/1(UnGatedMeasIndex)

== system Fusion_Frame_Model_Architecture/SENSOR_FUSION_SYSTEM/ROAD_GEOMETRY_CAMERA_FUSION/EGO_LANE_WIDTH_ESTIMATION ==
  EGO_LANE_WIDTH_prev : Inport
  EGO_LANE_RIGHT_LINE_TRACK : Inport  Port=2
  EGO_LANE_LEFT_LINE_TRACK : Inport  Port=3
  COMPUTE_SLOPE_AT_THE_POINTS : Subsystem
  COMPUTE_WIDTH_ALONG_THE_POINTS : Subsystem
  ESTIMATE_EGO_LANE_WIDTH : Subsystem
  INTERPOLATE_POINTS_ON_SMALLER_CURVE : Subsystem
  LOCATE_POINTS_WITH_SAME_SLOPE : Subsystem
  SELECT_CURVE_WITH_SMALLER_LENGTH : Subsystem
  EGO_LANE_WIDTH : Outport
  wires:
  EGO_LANE_RIGHT_LINE_TRACK/1 -> SELECT_CURVE_WITH_SMALLER_LENGTH/1(EGO_LANE_RIGHT_LINE_TRACK)
  EGO_LANE_LEFT_LINE_TRACK/1 -> SELECT_CURVE_WITH_SMALLER_LENGTH/2(EGO_LANE_LEFT_LINE_TRACK)
  SELECT_CURVE_WITH_SMALLER_LENGTH/1(SMALLER_CURVE) -> INTERPOLATE_POINTS_ON_SMALLER_CURVE/1(SMALLER_CURVE), COMPUTE_SLOPE_AT_THE_POINTS/1(SMALLER_CURVE)
  INTERPOLATE_POINTS_ON_SMALLER_CURVE/1(POINTS) -> COMPUTE_SLOPE_AT_THE_POINTS/2(POINTS), [points]
  SELECT_CURVE_WITH_SMALLER_LENGTH/2(LARGER_CURVE) -> LOCATE_POINTS_WITH_SAME_SLOPE/2(LARGER_CURVE)
  COMPUTE_SLOPE_AT_THE_POINTS/1(SLOPE) -> COMPUTE_WIDTH_ALONG_THE_POINTS/1(SLOPE), LOCATE_POINTS_WITH_SAME_SLOPE/1(SLOPE)
  LOCATE_POINTS_WITH_SAME_SLOPE/1(POINTS) -> COMPUTE_WIDTH_ALONG_THE_POINTS/3(POINTS_LARGER_CURVE)
  [points] -> COMPUTE_WIDTH_ALONG_THE_POINTS/2(POINTS_SMALLER_CURVE)
  COMPUTE_WIDTH_ALONG_THE_POINTS/1(WIDTH) -> ESTIMATE_EGO_LANE_WIDTH/2(WIDTH_Measurements)
  EGO_LANE_WIDTH_prev/1 -> ESTIMATE_EGO_LANE_WIDTH/1(WIDTH_prev)
  ESTIMATE_EGO_LANE_WIDTH/1(WIDTH_Upd) -> EGO_LANE_WIDTH/1

== system Fusion_Frame_Model_Architecture/SENSOR_FUSION_SYSTEM/ROAD_GEOMETRY_CAMERA_FUSION/ROAD_GEOMERY_AND_GRID_COMPUTATION ==
  EGO_LANE_WIDTH : Inport
  EGO_LANE_CENTER_LINE_TRACK : Inport  Port=2
  EGO_PARAM : Inport  Port=3
  ROAD_GRID_prev : Inport  Port=4
  COMPUTE_LEFT_LINE : Subsystem
  COMPUTE_NEXT_LEFT_LINE : Subsystem
  COMPUTE_NEXT_NEXT_LEFT_LINE : Subsystem
  COMPUTE_NEXT_NEXT_RIGHT_LINE : Subsystem
  COMPUTE_NEXT_RIGHT_LINE : Subsystem
  COMPUTE_OFFSET : Subsystem
  COMPUTE_OFFSET1 : Subsystem
  COMPUTE_OFFSET2 : Subsystem
  COMPUTE_OFFSET3 : Subsystem
  COMPUTE_OFFSET4 : Subsystem
  COMPUTE_OFFSET5 : Subsystem
  COMPUTE_RIGHT_LINE : Subsystem
  COMPUTE_ROAD_GRID : Subsystem
  SET_DATA : Subsystem
  ROAD_GEOMETRY : Outport
  ROAD_GRID : Outport  Port=2
  wires:
  COMPUTE_ROAD_GRID/1(GRID_Upd) -> ROAD_GRID/1
  EGO_LANE_WIDTH/1 -> COMPUTE_OFFSET3/1(Width), COMPUTE_OFFSET5/1(Width), COMPUTE_OFFSET4/1(Width), COMPUTE_OFFSET2/1(Width), COMPUTE_OFFSET1/1(Width), COMPUTE_OFFSET/1(Width)
  EGO_LANE_CENTER_LINE_TRACK/1 -> COMPUTE_RIGHT_LINE/1(EGO_LANE_CENTER_LINE_TRACK), COMPUTE_NEXT_RIGHT_LINE/1(EGO_LANE_CENTER_LINE_TRACK), COMPUTE_NEXT_NEXT_RIGHT_LINE/1(EGO_LANE_CENTER_LINE_TRACK), [C], COMPUTE_LEFT_LINE/2(EGO_LANE_CENTER_LINE_TRACK), COMPUTE_NEXT_LEFT_LINE/2(EGO_LANE_CENTER_LINE_TRACK), COMPUTE_NEXT_NEXT_LEFT_LINE/2(EGO_LANE_CENTER_LINE_TRACK)
  COMPUTE_OFFSET/1(Offset) -> COMPUTE_NEXT_NEXT_LEFT_LINE/1(OFFSET)
  COMPUTE_OFFSET1/1(Offset) -> COMPUTE_NEXT_LEFT_LINE/1(OFFSET)
  COMPUTE_OFFSET2/1(Offset) -> COMPUTE_LEFT_LINE/1(OFFSET)
  COMPUTE_OFFSET3/1(Offset) -> COMPUTE_NEXT_NEXT_RIGHT_LINE/2(OFFSET)
  COMPUTE_OFFSET4/1(Offset) -> COMPUTE_NEXT_RIGHT_LINE/2(OFFSET)
  COMPUTE_OFFSET5/1(Offset) -> COMPUTE_RIGHT_LINE/2(OFFSET)
  COMPUTE_NEXT_NEXT_LEFT_LINE/1(NNL) -> [NNL]
  COMPUTE_NEXT_LEFT_LINE/1(NL) -> [NL]
  COMPUTE_LEFT_LINE/1(L) -> [L]
  COMPUTE_NEXT_NEXT_RIGHT_LINE/1(NNR) -> [NNR]
  COMPUTE_NEXT_RIGHT_LINE/1(NR) -> [NR]
  COMPUTE_RIGHT_LINE/1(R) -> [R]
  EGO_PARAM/1 -> COMPUTE_ROAD_GRID/2(EGO_Param)
  [NNL] -> SET_DATA/1(EGO_LANE_NEXT_NEXT_LEFT_BOUNDARY)  "EGO_LANE_NEXT_NEXT_LEFT_BOUNDARY"
  [NL] -> SET_DATA/2(EGO_LANE_NEXT_LEFT_BOUNDARY)  "EGO_LANE_NEXT_LEFT_BOUNDARY"
  [L] -> SET_DATA/3(EGO_LANE_LEFT_BOUNDARY)  "EGO_LANE_LEFT_BOUNDARY"
  [C] -> SET_DATA/4(EGO_LANE_CENTER_TRACK_ESTIMATION)  "EGO_LANE_CENTER_TRACK_ESTIMATION"
  [R] -> SET_DATA/5(EGO_LANE_RIGHT_BOUNDARY)  "EGO_LANE_RIGHT_BOUNDARY"
  [NR] -> SET_DATA/6(EGO_LANE_NEXT_RIGHT_BOUNDARY)  "EGO_LANE_NEXT_RIGHT_BOUNDARY"
  [NNR] -> SET_DATA/7(EGO_LANE_NEXT_NEXT_RIGHT_BOUNDARY)  "EGO_LANE_NEXT_NEXT_RIGHT_BOUNDARY"
  SET_DATA/1(ROAD) -> [ROAD], ROAD_GEOMETRY/1
  [ROAD] -> COMPUTE_ROAD_GRID/1(RoadGeometry)
  ROAD_GRID_prev/1 -> COMPUTE_ROAD_GRID/3(GRID_Prev)

== system Fusion_Frame_Model_Architecture/SENSOR_FUSION_SYSTEM/ROAD_GEOMETRY_CAMERA_FUSION/SPATIAL_ALLIGNMENT_CLOTHOID_COEFFICIENTS ==
  CAM_SENSOR_PARAM : Inport
  LINE_CLOTHOID_MEASUREMENTS : Inport  Port=2
  CLUSTER_LINE_MEASUREMENTS : Subsystem
  SEGREGATE_LINE_MEASUREMENTS_AS_LEFT_AND_RIGHT_MEASUREMENTS : Subsystem
  SPATIAL_ALLIGNMENT_LINE_CLOTHOID_MEASUREMENTS : Subsystem
  TEMPORAL_ALLIGNMENT_LINE_CLOTHOID_MEASUREMENTS : Subsystem
  LEFT_LINE_MEAS : Outport
  "RIGHT_LINE_MEAS " : Outport  Port=2
  wires:
  CAM_SENSOR_PARAM/1 -> SPATIAL_ALLIGNMENT_LINE_CLOTHOID_MEASUREMENTS/1(CAM_SENSOR_PARAM)
  LINE_CLOTHOID_MEASUREMENTS/1 -> SPATIAL_ALLIGNMENT_LINE_CLOTHOID_MEASUREMENTS/2(LINE_CLOTHOID_MEASUREMENTS)
  SPATIAL_ALLIGNMENT_LINE_CLOTHOID_MEASUREMENTS/1(EGO_LANE_BOUNDARY_LINE_MEAS) -> TEMPORAL_ALLIGNMENT_LINE_CLOTHOID_MEASUREMENTS/1(EGO_LANE_BOUNDARY_LINE_MEAS_in)
  TEMPORAL_ALLIGNMENT_LINE_CLOTHOID_MEASUREMENTS/1(EGO_LANE_BOUNDARY_LINE_MEAS) -> SEGREGATE_LINE_MEASUREMENTS_AS_LEFT_AND_RIGHT_MEASUREMENTS/1(EGO_LANE_BOUNDARY_LINE_MEAS), CLUSTER_LINE_MEASUREMENTS/1(EGO_LANE_BOUNDARY_LINE_MEAS)
  CLUSTER_LINE_MEASUREMENTS/1(LINE_CLUSTERS) -> SEGREGATE_LINE_MEASUREMENTS_AS_LEFT_AND_RIGHT_MEASUREMENTS/2(LINE_CLUSTERS)
  SEGREGATE_LINE_MEASUREMENTS_AS_LEFT_AND_RIGHT_MEASUREMENTS/1(EGO_LANE_LEFT_BOUNDARY_LINE_MEAS) -> LEFT_LINE_MEAS/1
  SEGREGATE_LINE_MEASUREMENTS_AS_LEFT_AND_RIGHT_MEASUREMENTS/2(EGO_LANE_RIGHT_BOUNDARY_LINE_MEAS) -> "RIGHT_LINE_MEAS "/1

== system Fusion_Frame_Model_Architecture/SENSOR_MEASUREMENTS/RADAR_CAMERA_EGO_SENSOR_INTERFACE/CameraSensors ==
  time : Inport
  nObjCamera : Inport  Port=2
  CAMSensorBUS : Inport  Port=3  OutDataTypeStr=Bus: CameraMeasParam  PortDimensions=200  BusOutputAsStruct=on
  Camera1 : Subsystem  TreatAsAtomicUnit=on
  Camera2 : Subsystem  TreatAsAtomicUnit=on
  Camera3 : Subsystem  TreatAsAtomicUnit=on
  Camera4 : Subsystem  TreatAsAtomicUnit=on
  Camera5 : Subsystem  TreatAsAtomicUnit=on
  Camera6 : Subsystem  TreatAsAtomicUnit=on
  Camera7 : Subsystem  TreatAsAtomicUnit=on
  Camera8 : Subsystem  TreatAsAtomicUnit=on
  C1 : Outport
  C2 : Outport  Port=2
  C3 : Outport  Port=3
  C4 : Outport  Port=4
  C5 : Outport  Port=5
  C6 : Outport  Port=6
  C7 : Outport  Port=7
  C8 : Outport  Port=8
  wires:
  CAMSensorBUS/1 -> Camera1/3(SensorMeas), Camera2/3(SensorMeas), Camera3/3(SensorMeas), Camera4/3(SensorMeas), Camera6/3(SensorMeas), Camera8/3(SensorMeas), Camera7/3(SensorMeas), Camera5/3(SensorMeas)
  nObjCamera/1 -> Camera4/2(nObjCamera), Camera6/2(nObjCamera), Camera8/2(nObjCamera), Camera7/2(nObjCamera), Camera5/2(nObjCamera), Camera3/2(nObjCamera), Camera2/2(nObjCamera), Camera1/2(nObjCamera)
  Camera1/1(C1) -> C1/1
  time/1 -> Camera1/1(timeIdx), Camera4/1(timeIdx), Camera5/1(timeIdx), Camera6/1(timeIdx), Camera8/1(timeIdx), Camera7/1(timeIdx), Camera3/1(timeIdx), Camera2/1(timeIdx)
  Camera4/1(C4) -> C4/1
  Camera3/1(C3) -> C3/1
  Camera6/1(C6) -> C6/1
  Camera5/1(C5) -> C5/1
  Camera2/1(C2) -> C2/1
  Camera7/1(C7) -> C7/1
  Camera8/1(C8) -> C8/1

== system Fusion_Frame_Model_Architecture/SENSOR_MEASUREMENTS/RADAR_CAMERA_EGO_SENSOR_INTERFACE/Clock ==
  note: A n Array Of maximum number of sensor measurements for each Radar
  note: A n Array Of maximum number of sensor measurements for each Camera
  Add : Sum
  Constant : Constant
  Constant1 : Constant  Value=RAD_nMeas
  Constant2 : Constant  Value=CAM_nMeas
  Constant3 : Constant  Value=int32([2, 2, 2, 2, 2, 2, 2, 2])
  Data Type Conversion : DataTypeConversion  OutDataTypeStr=int16
  Digital Clock : DigitalClock  SampleTime=SamplingTime
  Gain : Gain  Gain=1/SamplingTime
  time : Outport
  nObjRadar : Outport  Port=2
  nObjCamera : Outport  Port=3
  nLinesCamera : Outport  Port=4
  wires:
  Digital Clock/1 -> Gain/1
  Gain/1 -> Add/1
  Add/1 -> Data Type Conversion/1
  Constant/1 -> Add/2
  Data Type Conversion/1 -> time/1
  Constant1/1 -> nObjRadar/1
  Constant2/1 -> nObjCamera/1
  Constant3/1 -> nLinesCamera/1

== system Fusion_Frame_Model_Architecture/SENSOR_MEASUREMENTS/RADAR_CAMERA_EGO_SENSOR_INTERFACE/EgoSensors ==
  timeIdx : Inport
  In1 : Inport  Port=2  OutDataTypeStr=Bus: EGO_PARAM  PortDimensions=1
  Assignment : Assignment  DiagnosticForDimensions=Warning  IndexOptions=Index vector (dialog)  Indices=1  OutputSizes=1
  Bus Creator : BusCreator  Inputs=7  OutDataTypeStr=Bus: EGO_PARAM  NonVirtualBus=on
      settings: InheritFromInputs=off
  ExtractMeasParam : Subsystem
  EgoSensorData : Outport
  EgoIgnitionStatus : Outport  Port=2
  wires:
  timeIdx/1 -> ExtractMeasParam/1(timeIdx)
  Bus Creator/1 -> Assignment/2
  Assignment/1 -> EgoSensorData/1
  ExtractMeasParam/1(EgoTimeStamp) -> Bus Creator/1  "TimeStamp"
  ExtractMeasParam/2(EgoPx) -> Bus Creator/2  "px"
  ExtractMeasParam/3(EgoPy) -> Bus Creator/3  "py"
  ExtractMeasParam/4(EgoVx) -> Bus Creator/4  "vx"
  ExtractMeasParam/6(EgoYaw) -> Bus Creator/6  "yaw"
  ExtractMeasParam/7(EgoYawRate) -> Bus Creator/7  "yawRate"
  ExtractMeasParam/5(EgoVy) -> Bus Creator/5  "vy"
  In1/1 -> Assignment/1
  ExtractMeasParam/8(EgoIgnitionStatus) -> EgoIgnitionStatus/1

== system Fusion_Frame_Model_Architecture/SENSOR_MEASUREMENTS/RADAR_CAMERA_EGO_SENSOR_INTERFACE/RadarSensors ==
  time : Inport
  nObjRadar : Inport  Port=2
  RADSensorBUS : Inport  Port=3  OutDataTypeStr=Bus: RadarMeasParam  PortDimensions=200  BusOutputAsStruct=on
  Radar1 : Subsystem  TreatAsAtomicUnit=on
  Radar2 : Subsystem  TreatAsAtomicUnit=on
  Radar3 : Subsystem  TreatAsAtomicUnit=on
  Radar4 : Subsystem  TreatAsAtomicUnit=on
  Radar5 : Subsystem  TreatAsAtomicUnit=on
  Radar6 : Subsystem  TreatAsAtomicUnit=on
  R1 : Outport
  R2 : Outport  Port=2
  R3 : Outport  Port=3
  R4 : Outport  Port=4
  R5 : Outport  Port=5
  R6 : Outport  Port=6
  wires:
  RADSensorBUS/1 -> Radar2/3(SensorMeas), Radar6/3(SensorMeas), Radar5/3(SensorMeas), Radar4/3(SensorMeas), Radar3/3(SensorMeas), Radar1/3(SensorMeas)
  nObjRadar/1 -> Radar3/2(nObjRadar), Radar6/2(nObjRadar), Radar5/2(nObjRadar), Radar4/2(nObjRadar), Radar2/2(nObjRadar), Radar1/2(nObjRadar)
  Radar1/1(R1) -> R1/1
  time/1 -> Radar3/1(timeIdx), Radar6/1(timeIdx), Radar5/1(timeIdx), Radar4/1(timeIdx), Radar2/1(timeIdx), Radar1/1(timeIdx)
  Radar4/1(R4) -> R4/1
  Radar3/1(R3) -> R3/1
  Radar6/1(R6) -> R6/1
  Radar5/1(R5) -> R5/1
  Radar2/1(R2) -> R2/1

== system Fusion_Frame_Model_Architecture/SENSOR_MEASUREMENTS/RADAR_CAMERA_EGO_SENSOR_INTERFACE/RoadSensors ==
  time : Inport
  nLinesCamera : Inport  Port=2
  CameraLineCoeff1 : Inport  Port=3  OutDataTypeStr=Bus: LineMeasParam  PortDimensions=10
  Camera1 : Subsystem  TreatAsAtomicUnit=on
  Camera2 : Subsystem  TreatAsAtomicUnit=on
  Camera3 : Subsystem  TreatAsAtomicUnit=on
  Camera4 : Subsystem  TreatAsAtomicUnit=on
  Camera5 : Subsystem  TreatAsAtomicUnit=on
  Camera6 : Subsystem  TreatAsAtomicUnit=on
  Camera7 : Subsystem  TreatAsAtomicUnit=on
  Camera8 : Subsystem  TreatAsAtomicUnit=on
  C1 : Outport
  C2 : Outport  Port=2
  C3 : Outport  Port=3
  C4 : Outport  Port=4
  C5 : Outport  Port=5
  C6 : Outport  Port=6
  C7 : Outport  Port=7
  C8 : Outport  Port=8
  wires:
  Camera2/1(C1) -> C2/1
  Camera7/1(C1) -> C7/1
  CameraLineCoeff1/1 -> Camera1/3(CameraLineCoeff), Camera2/3(CameraLineCoeff), Camera3/3(CameraLineCoeff), Camera4/3(CameraLineCoeff), Camera5/3(CameraLineCoeff), Camera6/3(CameraLineCoeff), Camera8/3(CameraLineCoeff), Camera7/3(CameraLineCoeff)
  time/1 -> Camera1/1(timeIdx), Camera2/1(timeIdx), Camera3/1(timeIdx), Camera4/1(timeIdx), Camera5/1(timeIdx), Camera6/1(timeIdx), Camera8/1(timeIdx), Camera7/1(timeIdx)
  Camera1/1(C1) -> C1/1
  Camera6/1(C1) -> C6/1
  Camera5/1(C1) -> C5/1
  Camera8/1(C1) -> C8/1
  nLinesCamera/1 -> Camera2/2(nLines), Camera3/2(nLines), Camera4/2(nLines), Camera5/2(nLines), Camera6/2(nLines), Camera8/2(nLines), Camera7/2(nLines), Camera1/2(nLines)
  Camera3/1(C1) -> C3/1
  Camera4/1(C1) -> C4/1

== system Fusion_Frame_Model_Architecture/SENSOR_FUSION_SYSTEM/OBJECT_TRACKER_SENSOR_FUSION/CAMERA_HOMOGENEOUS_FUSION/DATA_ASSOCIATION_AND_ESTIMATION ==
  GatedMeasFlag : Inport
  MeasLogLikelihood : Inport  Port=2
  Meas : Inport  Port=3
  CAM_PARAM : Inport  Port=4
  TrackParamPred : Inport  Port=5
  Terminator{,1..3} (4 alike) : Terminator
  TrackParamUpd : Outport
  wires:
  Meas/1 -> Terminator2/1
  MeasLogLikelihood/1 -> Terminator1/1
  GatedMeasFlag/1 -> Terminator/1
  TrackParamPred/1 -> TrackParamUpd/1
  CAM_PARAM/1 -> Terminator3/1

== system Fusion_Frame_Model_Architecture/SENSOR_FUSION_SYSTEM/OBJECT_TRACKER_SENSOR_FUSION/CAMERA_HOMOGENEOUS_FUSION/GATING ==
  MEAS : Inport
  CAMERA_CLUSTERS : Inport  Port=2
  CAM_PARAM : Inport  Port=3
  TrackParamPred : Inport  Port=4
  FIND_UNASSOCIATED_CLUSTERS : Subsystem
  GET_DATA : Subsystem
  MEASUREMENT_TO_TRACK_GATING_AND_LOGLIKELIHOOD_COMPUTATION : Subsystem
  RESOLVE_GATING_AMBIGUITY : Subsystem
  GatedMeasFlag : Outport
  GatedMeasLogLikelihood : Outport  Port=2
  UnGatedMeasCluster : Outport  Port=3
  wires:
  MEAS/1 -> MEASUREMENT_TO_TRACK_GATING_AND_LOGLIKELIHOOD_COMPUTATION/4(Meas), FIND_UNASSOCIATED_CLUSTERS/3(measCLUSTERS)
  MEASUREMENT_TO_TRACK_GATING_AND_LOGLIKELIHOOD_COMPUTATION/2(GatedMeasFlagArray) -> RESOLVE_GATING_AMBIGUITY/3(GatedMeasFlagArrayIn)
  MEASUREMENT_TO_TRACK_GATING_AND_LOGLIKELIHOOD_COMPUTATION/3(GatedMeasLogLikelihood) -> RESOLVE_GATING_AMBIGUITY/4(GatedMeasLogLikelihoodIn)
  TrackParamPred/1 -> GET_DATA/1(TRACKS)
  GET_DATA/1(nTracksPred) -> RESOLVE_GATING_AMBIGUITY/1(nTracks), MEASUREMENT_TO_TRACK_GATING_AND_LOGLIKELIHOOD_COMPUTATION/1(nTracks)
  GET_DATA/2(TrackParam) -> MEASUREMENT_TO_TRACK_GATING_AND_LOGLIKELIHOOD_COMPUTATION/2(TrackParamPred)
  MEASUREMENT_TO_TRACK_GATING_AND_LOGLIKELIHOOD_COMPUTATION/1(nMeas) -> RESOLVE_GATING_AMBIGUITY/2(nMeas)
  RESOLVE_GATING_AMBIGUITY/1(GatedMeasFlagArray) -> GatedMeasFlag/1, FIND_UNASSOCIATED_CLUSTERS/1(GatedMeasFlagArray)
  CAMERA_CLUSTERS/1 -> FIND_UNASSOCIATED_CLUSTERS/2(Clusters)
  RESOLVE_GATING_AMBIGUITY/2(GatedMeasLogLikelihood) -> GatedMeasLogLikelihood/1
  FIND_UNASSOCIATED_CLUSTERS/1(UngatedCLUSTERS) -> UnGatedMeasCluster/1
  CAM_PARAM/1 -> MEASUREMENT_TO_TRACK_GATING_AND_LOGLIKELIHOOD_COMPUTATION/3(SnsrParam)

== system Fusion_Frame_Model_Architecture/SENSOR_FUSION_SYSTEM/OBJECT_TRACKER_SENSOR_FUSION/CAMERA_HOMOGENEOUS_FUSION/NEAREST_NEIGHBOUR_CLUSTERING_FOR_CAMERA_MEASUREMENT ==
  CAMERA_MEAS : Inport
  GET_NUM_OF_MEAS : Subsystem
  NN_MEASUREMENT_GROUPING_WITHIN_EPS : Subsystem  TreatAsAtomicUnit=on
  CAMERA_CLUSTERS : Outport
  wires:
  GET_NUM_OF_MEAS/1(nMeas) -> NN_MEASUREMENT_GROUPING_WITHIN_EPS/1(nMeas)
  CAMERA_MEAS/1 -> GET_NUM_OF_MEAS/1(CAM_MEAS_CTS), NN_MEASUREMENT_GROUPING_WITHIN_EPS/2(Meas)
  NN_MEASUREMENT_GROUPING_WITHIN_EPS/1(CAMERA_CLUSTERS) -> CAMERA_CLUSTERS/1

== system Fusion_Frame_Model_Architecture/SENSOR_FUSION_SYSTEM/OBJECT_TRACKER_SENSOR_FUSION/CAMERA_HOMOGENEOUS_FUSION/STATE_PREDICTION ==
  TrackParamPrev : Inport
  GET_DATA : Subsystem
  SET_DATA : Subsystem
  TRACK_STATE_PREDICTION : Subsystem
  Unit Delay : UnitDelay  InitialCondition=TRACK_EST_RAD_INIT  SampleTime=-1
  TrackParamPred : Outport
  wires:
  TrackParamPrev/1 -> Unit Delay/1
  Unit Delay/1 -> GET_DATA/1(TRACKS), SET_DATA/1(TRACKS_in)
  GET_DATA/1(nTracksPrev) -> TRACK_STATE_PREDICTION/1(nTracks)
  GET_DATA/2(TrackParam) -> TRACK_STATE_PREDICTION/2(TrackParamPred)
  TRACK_STATE_PREDICTION/1(StatePredBus) -> SET_DATA/2(TrackParam)
  SET_DATA/1(TRACKS) -> TrackParamPred/1

== system Fusion_Frame_Model_Architecture/SENSOR_FUSION_SYSTEM/OBJECT_TRACKER_SENSOR_FUSION/CAMERA_HOMOGENEOUS_FUSION/TRACK_MANAGER ==
  TrackParamIn : Inport
  UnGatedClusters : Inport  Port=2
  Grid : Inport  Port=3
  Bus Creator : BusCreator  Inputs=6  OutDataTypeStr=Bus: TRACK_ESTIMATES_BUS  NonVirtualBus=on
      settings: InheritFromInputs=off
  Bus Selector : BusSelector  OutputSignals=nValidTracks,TrackParam,TrackIDList,IsTrackIDused,FirstAvailableIDindex,LastAvailableIDindex
  Terminator : Terminator
  Terminator1 : Terminator
  TrackParamUpd : Outport
  wires:
  UnGatedClusters/1 -> Terminator/1
  Bus Creator/1 -> TrackParamUpd/1
  Bus Selector/4 -> Bus Creator/4  "<IsTrackIDused>"
  Bus Selector/2 -> Bus Creator/2  "<TrackParam>"
  Bus Selector/3 -> Bus Creator/3  "<TrackIDList>"
  TrackParamIn/1 -> Bus Selector/1
  Bus Selector/1 -> Bus Creator/1  "<nValidTracks>"
  Bus Selector/5 -> Bus Creator/5  "<FirstAvailableIDindex>"
  Bus Selector/6 -> Bus Creator/6  "<LastAvailableIDindex>"
  Grid/1 -> Terminator1/1

== system Fusion_Frame_Model_Architecture/SENSOR_FUSION_SYSTEM/OBJECT_TRACKER_SENSOR_FUSION/RADAR_CAMERA_HETEROGENEOUS_FUSION/FORM_TRACK_GROUPS ==
  RAD_TRACKS : Inport
  RAD_CAM_FUSED_TRACKS : Inport  Port=2
  CAM_TRACKS : Inport  Port=3
  Ground : Ground
  Terminator : Terminator
  Terminator1 : Terminator
  Terminator2 : Terminator
  GROUPED_TRACKS_IDs : Outport
  wires:
  RAD_CAM_FUSED_TRACKS/1 -> Terminator/1
  RAD_TRACKS/1 -> Terminator1/1
  CAM_TRACKS/1 -> Terminator2/1
  Ground/1 -> GROUPED_TRACKS_IDs/1

== system Fusion_Frame_Model_Architecture/SENSOR_FUSION_SYSTEM/OBJECT_TRACKER_SENSOR_FUSION/RADAR_CAMERA_HETEROGENEOUS_FUSION/STATE_PREDICTION ==
  RAD_CAM_TRACKS_PREV : Inport
  Unit Delay1 : UnitDelay  InitialCondition=TRACK_EST_FUS_INIT  SampleTime=-1
  RAD_CAM_TRACKS_PRED : Outport
  wires:
  RAD_CAM_TRACKS_PREV/1 -> Unit Delay1/1
  Unit Delay1/1 -> RAD_CAM_TRACKS_PRED/1

== system Fusion_Frame_Model_Architecture/SENSOR_FUSION_SYSTEM/OBJECT_TRACKER_SENSOR_FUSION/RADAR_CAMERA_HETEROGENEOUS_FUSION/TRACK_MANAGER ==
  RAD_CAM_FUSED_TRACKS : Inport
  RAD_TRACKS : Inport  Port=2
  CAM_TRACKS : Inport  Port=3
  Bus Creator : BusCreator  Inputs=6  OutDataTypeStr=Bus: TRACK_ESTIMATES_BUS  NonVirtualBus=on
      settings: InheritFromInputs=off
  Bus Selector : BusSelector  OutputSignals=nValidTracks,TrackParam,TrackIDList,IsTrackIDused,FirstAvailableIDindex,LastAvailableIDindex
  Terminator : Terminator
  Terminator1 : Terminator
  RAD_CAM_TRACKS_FUS : Outport
  wires:
  RAD_TRACKS/1 -> Terminator/1
  Bus Selector/4 -> Bus Creator/4  "<IsTrackIDused>"
  Bus Selector/2 -> Bus Creator/2  "<TrackParam>"
  Bus Selector/3 -> Bus Creator/3  "<TrackIDList>"
  RAD_CAM_FUSED_TRACKS/1 -> Bus Selector/1
  Bus Selector/1 -> Bus Creator/1  "<nValidTracks>"
  Bus Selector/5 -> Bus Creator/5  "<FirstAvailableIDindex>"
  Bus Selector/6 -> Bus Creator/6  "<LastAvailableIDindex>"
  Bus Creator/1 -> RAD_CAM_TRACKS_FUS/1
  CAM_TRACKS/1 -> Terminator1/1

== system Fusion_Frame_Model_Architecture/SENSOR_FUSION_SYSTEM/OBJECT_TRACKER_SENSOR_FUSION/RADAR_CAMERA_HETEROGENEOUS_FUSION/TRACK_TO_TRACK_FUSION ==
  GROUPED_TRACKS_IDs : Inport
  RAD_TRACKS : Inport  Port=2
  CAM_TRACKS : Inport  Port=3
  RAD_CAM_FUSED_TRACKS_PRED : Inport  Port=4
  Terminator1 : Terminator
  Terminator2 : Terminator
  Terminator3 : Terminator
  RAD_CAM_FUSED_TRACKS_UPD : Outport
  wires:
  RAD_TRACKS/1 -> Terminator1/1
  CAM_TRACKS/1 -> Terminator2/1
  GROUPED_TRACKS_IDs/1 -> Terminator3/1
  RAD_CAM_FUSED_TRACKS_PRED/1 -> RAD_CAM_FUSED_TRACKS_UPD/1

== system Fusion_Frame_Model_Architecture/SENSOR_FUSION_SYSTEM/OBJECT_TRACKER_SENSOR_FUSION/RADAR_HOMOGENEOUS_FUSION/DATA_ASSOCIATION_AND_ESTIMATION ==
  GatedMeasFlag : Inport
  MeasLogLikelihood : Inport  Port=2
  Meas : Inport  Port=3
  RAD_PARAM : Inport  Port=4
  TrackParamPred : Inport  Port=5
  Terminator{,1..3} (4 alike) : Terminator
  TrackParamUpd : Outport
  wires:
  Meas/1 -> Terminator2/1
  MeasLogLikelihood/1 -> Terminator1/1
  GatedMeasFlag/1 -> Terminator/1
  TrackParamPred/1 -> TrackParamUpd/1
  RAD_PARAM/1 -> Terminator3/1
